simulink model "testIssLVLHPointingModel"  (R2023b)
settings: Solver=ode4  StartTime=0  StopTime=tFinal  FixedStep=dtSim  RelTol=1e-3
values from neighbouring files (symbols this model uses):
  dtSim = 0.1    [test01IssLVLHPointing.m]    (also in test02IssLVLHPointing.m)
libraries: orbitProp2B_sl x1, issLVLHPointingSim_sl x1
settings Model: Creator=gilbu  LastModifiedBy=gilbu

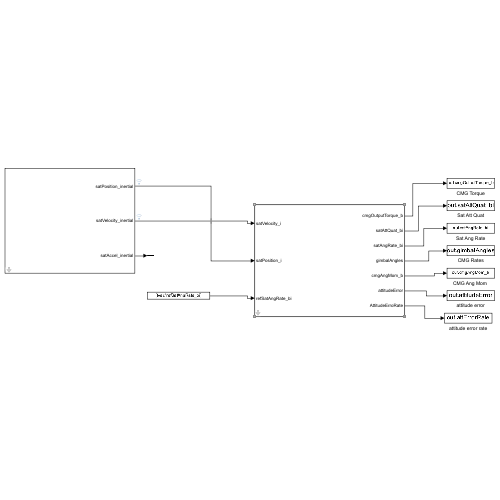
[thumbnail: Simulink's stored preview of the top-level diagram]
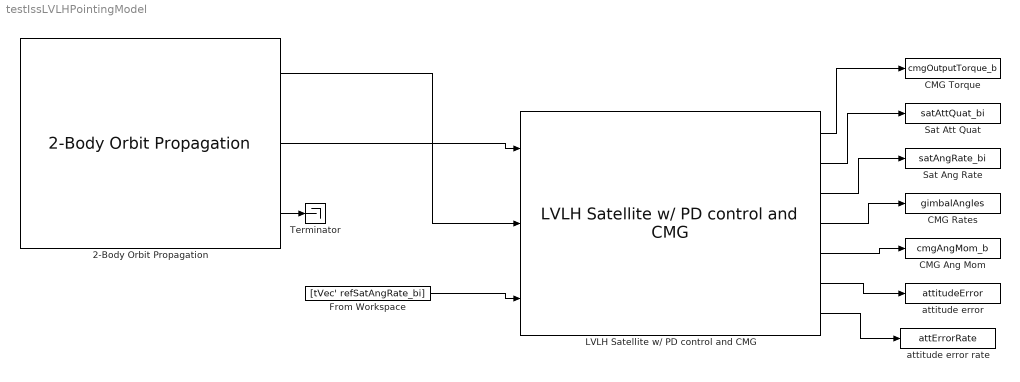
== system testIssLVLHPointingModel ==
  2-Body Orbit Propagation : orbitProp2B_sl/2-Body Orbit Propagation  mu=mu  satPosition0=satPosition0  satVelocity0=satVelocity0
  "CMG Ang Mom " : ToWorkspace  VariableName=cmgAngMom_b  SaveFormat=Timeseries  SampleTime=dtSim
  CMG Rates : ToWorkspace  VariableName=gimbalAngles  SaveFormat=Timeseries  SampleTime=dtSim
  CMG Torque : ToWorkspace  VariableName=cmgOutputTorque_b  SaveFormat=Timeseries  SampleTime=dtSim
  From Workspace : FromWorkspace  VariableName=[tVec' refSatAngRate_bi]  SampleTime=dtSim
  LVLH Satellite w/ PD control and CMG : issLVLHPointingSim_sl/LVLH Satellite w// PD control and CMG  adcsParams=adcsParams  hwParams=hwParams  satDynParams=satDynParams
      link override ADCS- TRIAD-PD Controller: rotorAngRate=hwParams.rotorAngRate  maxGimbalRate=hwParams.maxGimbalRates  innerAngDistGain=adcsParams.innerAngDistGain  outerAngDistGain=adcsParams.outerAngDistGain  satInertiaTensor=satDynParams.satInertiaTensor
      link override Sensor Hardware/Gimbal Rate Measurments: gimbalErrorFlag=hwParams.gimbalErrorFlag  gimbalBias=hwParams.gimbalBias  gimbalNoisePower=hwParams.gimbalNoisePower
  Sat Ang Rate : ToWorkspace  VariableName=satAngRate_bi  SaveFormat=Timeseries  SampleTime=dtSim
  Sat Att Quat : ToWorkspace  VariableName=satAttQuat_bi  SaveFormat=Timeseries  SampleTime=dtSim
  Terminator : Terminator
  attitude error : ToWorkspace  VariableName=attitudeError  SaveFormat=Timeseries  SampleTime=dtSim
  attitude error rate : ToWorkspace  VariableName=attErrorRate  SaveFormat=Timeseries  SampleTime=dtSim
  wires:
  LVLH Satellite w/ PD control and CMG/1 -> CMG Torque/1
  LVLH Satellite w/ PD control and CMG/2 -> Sat Att Quat/1
  LVLH Satellite w/ PD control and CMG/3 -> Sat Ang Rate/1
  LVLH Satellite w/ PD control and CMG/4 -> CMG Rates/1
  LVLH Satellite w/ PD control and CMG/5 -> "CMG Ang Mom "/1
  2-Body Orbit Propagation/2 -> LVLH Satellite w/ PD control and CMG/1
  2-Body Orbit Propagation/1 -> LVLH Satellite w/ PD control and CMG/2
  2-Body Orbit Propagation/3 -> Terminator/1
  From Workspace/1 -> LVLH Satellite w/ PD control and CMG/3
  LVLH Satellite w/ PD control and CMG/6 -> attitude error/1
  LVLH Satellite w/ PD control and CMG/7 -> attitude error rate/1
